simulink model "Ballbot_System_LQR"  (R2020b)
settings: Solver=VariableStepAuto  StartTime=0.0  StopTime=30  RelTol=1e-3
values from neighbouring files (symbols this model uses):
  a_d = 0.8    [SYSTEM_BALLBOT.m]
  a_gc = 0.8    [SYSTEM_BALLBOT.m]
  a_gd = 0.999    [SYSTEM_BALLBOT.m]
  BATTERY = 8000    [SYSTEM_BALLBOT.m]
  GYRO0 = 600    [SYSTEM_BALLBOT.m]
  k_f = K_lqr(1:4)    [SYSTEM_BALLBOT.m]
  pwm_gain = 1    [SYSTEM_BALLBOT.m]
  pwm_offset = 0    [SYSTEM_BALLBOT.m]
  TIME_START = 100    [SYSTEM_BALLBOT.m]
  TS = 0.004    [SYSTEM_BALLBOT.m]
  ts1 = 0.004    [SYSTEM_BALLBOT.m]
  XIV = [ ... (first row only)    [SYSTEM_BALLBOT.m]
undefined symbols (not defined in the file or in its folder): A, B, C, D, Rs, Rw
libraries: legoev3lib x9, simulink x3
settings Model: Creator=ADMIN  LastModifiedBy=ADMIN
settings DebuggingCC: UnconnectedInputMsg=none  UnconnectedOutputMsg=none  UnconnectedLineMsg=none
settings ModelReferenceCC: EnableRefExpFcnMdlSchedulingChecks=off
settings RTWCC: GPUComputeCapability=5.0
settings ConfigComp: CovBoundaryAbsTol=1.0e-5

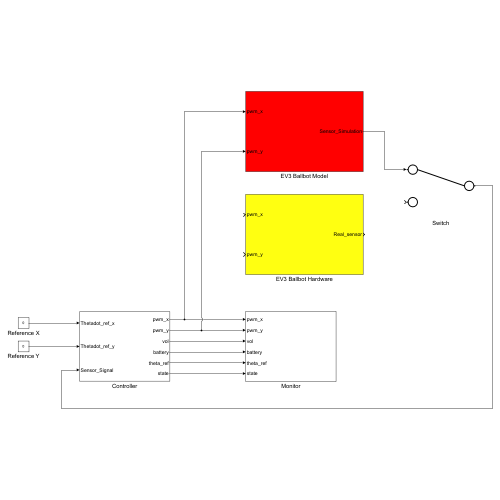
[thumbnail: Simulink's stored preview of the top-level diagram]
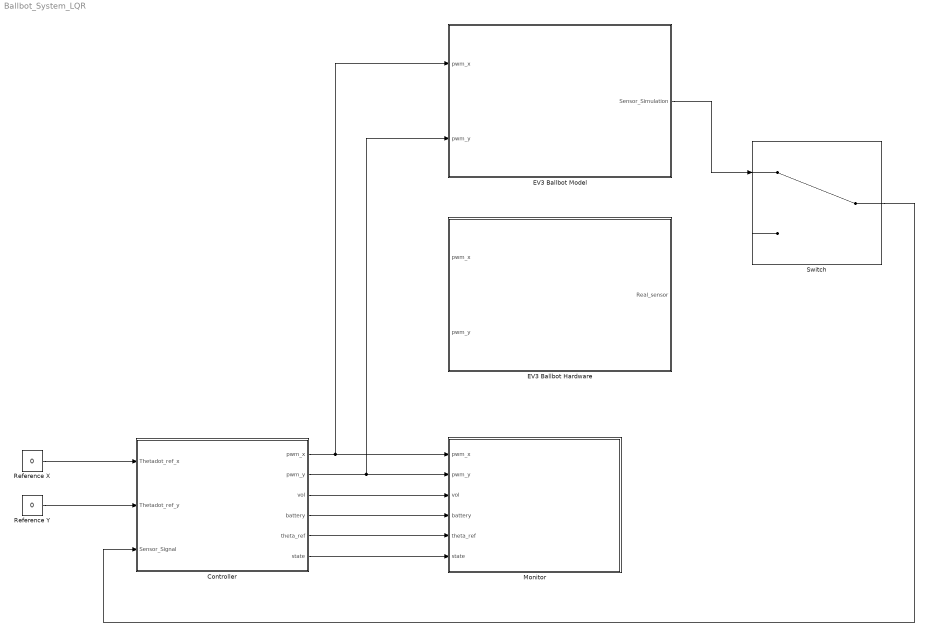
== system Ballbot_System_LQR ==
  Controller : Subsystem
  EV3 Ballbot Hardware : Subsystem
  EV3 Ballbot Model : Subsystem
  Monitor : Subsystem
  Reference X : Constant  Value=0
  Reference Y : Constant  Value=0
  Switch : ManualSwitch
  wires:
  Controller/1(pwm_x) -> EV3 Ballbot Model/1(pwm_x), Monitor/1(pwm_x)
  Controller/4(battery) -> Monitor/4(battery)
  Controller/6(state) -> Monitor/6(state)
  EV3 Ballbot Model/1(Sensor_Simulation) -> Switch/1
  Controller/5(theta_ref) -> Monitor/5(theta_ref)
  Switch/1 -> Controller/3(Sensor_Signal)
  Controller/3(vol) -> Monitor/3(vol)
  Reference Y/1 -> Controller/2(Thetadot_ref_y)
  Controller/2(pwm_y) -> EV3 Ballbot Model/2(pwm_y), Monitor/2(pwm_y)
  Reference X/1 -> Controller/1(Thetadot_ref_x)

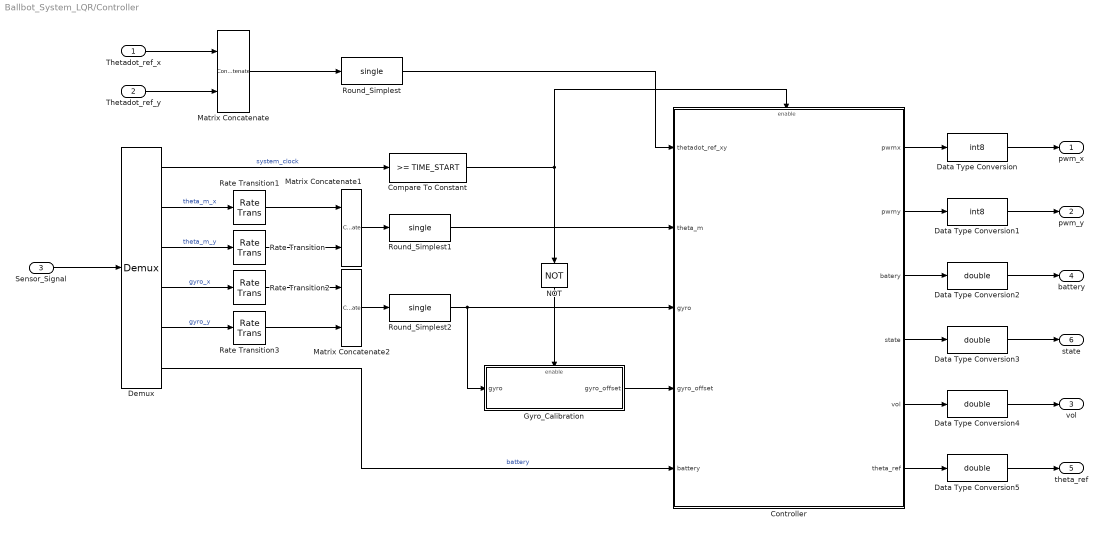
== system Ballbot_System_LQR/Controller ==
  Thetadot_ref_x : Inport
  Thetadot_ref_y : Inport  Port=2
  Sensor_Signal : Inport  Port=3
  Compare To Constant : simulink/Logic and Bit Operations/Compare To Constant  relop=>=  const=TIME_START  OutDataTypeStr=boolean
  Controller : Subsystem
  Data Type Conversion : DataTypeConversion  OutDataTypeStr=int8  RndMeth=Simplest
  Data Type Conversion1 : DataTypeConversion  OutDataTypeStr=int8  RndMeth=Simplest
  Data Type Conversion{2..5} (4 alike) : DataTypeConversion  OutDataTypeStr=double  RndMeth=Simplest
  Demux : Demux  Outputs=6
      settings: DisplayOption=none
  Gyro_Calibration : Subsystem
  Matrix Concatenate : Concatenate  Mode=Multidimensional array  ConcatenateDimension=2
  Matrix Concatenate1 : Concatenate  Mode=Multidimensional array  ConcatenateDimension=2
  Matrix Concatenate2 : Concatenate  Mode=Multidimensional array  ConcatenateDimension=2
  NOT : Logic  Operator=NOT  IconShape=distinctive  AllPortsSameDT=off  OutDataTypeStr=boolean
  Rate Transition{,1..3} (4 alike) : RateTransition  OutPortSampleTime=TS
  Round_Simplest : DataTypeConversion  OutDataTypeStr=single  RndMeth=Round
  Round_Simplest1 : DataTypeConversion  OutDataTypeStr=single  RndMeth=Round
  Round_Simplest2 : DataTypeConversion  OutDataTypeStr=single  RndMeth=Round
  pwm_x : Outport
  pwm_y : Outport  Port=2
  vol : Outport  Port=3
  battery : Outport  Port=4
  theta_ref : Outport  Port=5
  state : Outport  Port=6
  wires:
  Thetadot_ref_x/1 -> Matrix Concatenate/1
  Thetadot_ref_y/1 -> Matrix Concatenate/2
  Matrix Concatenate/1 -> Round_Simplest/1
  Sensor_Signal/1 -> Demux/1
  Demux/3 -> Rate Transition/1  "theta_m_y"
  Matrix Concatenate1/1 -> Round_Simplest1/1
  Matrix Concatenate2/1 -> Round_Simplest2/1
  Demux/1 -> Compare To Constant/1  "system_clock"
  Compare To Constant/1 -> Controller/Enable, NOT/1
  Round_Simplest2/1 -> Controller/3(gyro), Gyro_Calibration/1(gyro)
  NOT/1 -> Gyro_Calibration/Enable
  Demux/6 -> Controller/5(battery)  "battery"
  Gyro_Calibration/1(gyro_offset) -> Controller/4(gyro_offset)
  Round_Simplest1/1 -> Controller/2(theta_m)
  Round_Simplest/1 -> Controller/1(thetadot_ref_xy)
  Controller/1(pwmx) -> Data Type Conversion/1
  Data Type Conversion/1 -> pwm_x/1
  Data Type Conversion1/1 -> pwm_y/1
  Controller/2(pwmy) -> Data Type Conversion1/1
  Data Type Conversion2/1 -> battery/1
  Controller/3(batery) -> Data Type Conversion2/1
  Data Type Conversion3/1 -> state/1
  Controller/4(state) -> Data Type Conversion3/1
  Data Type Conversion4/1 -> vol/1
  Controller/5(vol) -> Data Type Conversion4/1
  Data Type Conversion5/1 -> theta_ref/1
  Controller/6(theta_ref) -> Data Type Conversion5/1
  Rate Transition/1 -> Matrix Concatenate1/2
  Rate Transition1/1 -> Matrix Concatenate1/1
  Demux/4 -> Rate Transition2/1  "gyro_x"
  Rate Transition2/1 -> Matrix Concatenate2/1
  Demux/2 -> Rate Transition1/1  "theta_m_x"
  Rate Transition3/1 -> Matrix Concatenate2/2
  Demux/5 -> Rate Transition3/1  "gyro_y"

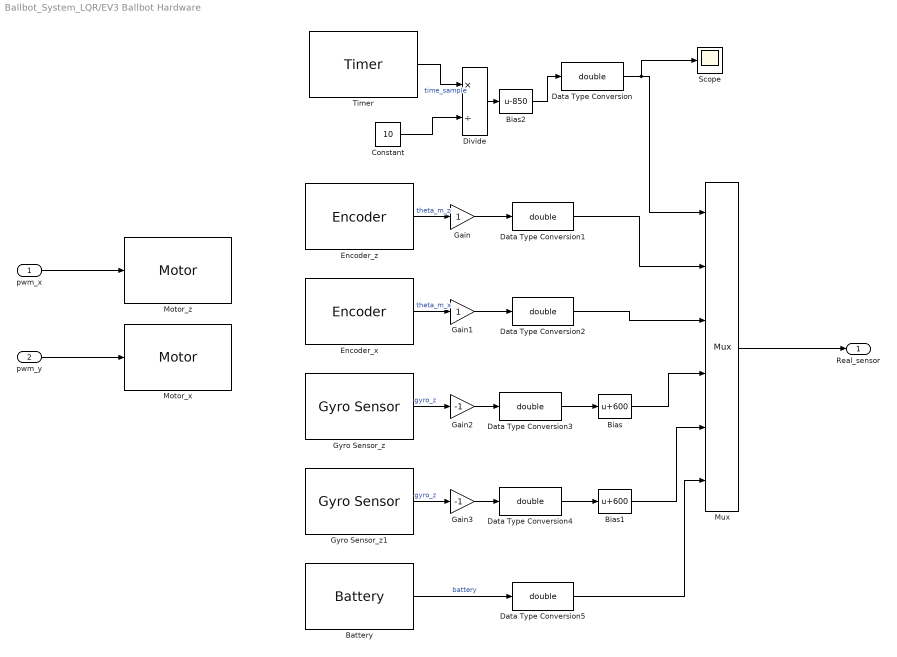
== system Ballbot_System_LQR/EV3 Ballbot Hardware ==
  pwm_x : Inport
  pwm_y : Inport  Port=2
  Battery : legoev3lib/Battery  SampleTime=TS
  Bias : Bias  Bias=600
  Bias1 : Bias  Bias=600
  Bias2 : Bias  Bias=-850
  Constant : Constant  Value=10
  Data Type Conversion{,1..5} (6 alike) : DataTypeConversion  OutDataTypeStr=double  RndMeth=Nearest
  Divide : Product  Inputs=*/
  Encoder_x : legoev3lib/Encoder  portNumber=C  opMode=Reset by external signal  sampleTime=TS
  Encoder_z : legoev3lib/Encoder  portNumber=B  opMode=Reset by external signal  sampleTime=TS
  Gain : Gain
  Gain1 : Gain
  Gain2 : Gain  Gain=-1
  Gain3 : Gain  Gain=-1
  Gyro Sensor_z : legoev3lib/Gyro Sensor  portNumber=2  sampleTime=TS
  Gyro Sensor_z1 : legoev3lib/Gyro Sensor  portNumber=3  sampleTime=TS
  Motor_x : legoev3lib/Motor  sportNumber=C  sstopAction=Brake
  Motor_z : legoev3lib/Motor  sportNumber=B  sstopAction=Brake
  Mux : Mux  Inputs=6
      settings: DisplayOption=signals
  Scope : Scope
  Timer : legoev3lib/Timer  SampleTime=TS
  Real_sensor : Outport
  wires:
  pwm_x/1 -> Motor_z/1
  pwm_y/1 -> Motor_x/1
  Timer/1 -> Divide/1  "time_sample"
  Encoder_z/1 -> Gain/1  "theta_m_z"
  Encoder_x/1 -> Gain1/1  "theta_m_x"
  Battery/1 -> Data Type Conversion5/1  "battery"
  Data Type Conversion/1 -> Scope/1, Mux/1
  Data Type Conversion1/1 -> Mux/2
  Data Type Conversion2/1 -> Mux/3
  Data Type Conversion5/1 -> Mux/6
  Mux/1 -> Real_sensor/1
  Gain/1 -> Data Type Conversion1/1
  Gain1/1 -> Data Type Conversion2/1
  Gain2/1 -> Data Type Conversion3/1
  Gyro Sensor_z/1 -> Gain2/1  "gyro_z"
  Gyro Sensor_z1/1 -> Gain3/1  "gyro_z"
  Gain3/1 -> Data Type Conversion4/1
  Data Type Conversion3/1 -> Bias/1
  Data Type Conversion4/1 -> Bias1/1
  Bias/1 -> Mux/4
  Bias1/1 -> Mux/5
  Constant/1 -> Divide/2
  Divide/1 -> Bias2/1
  Bias2/1 -> Data Type Conversion/1

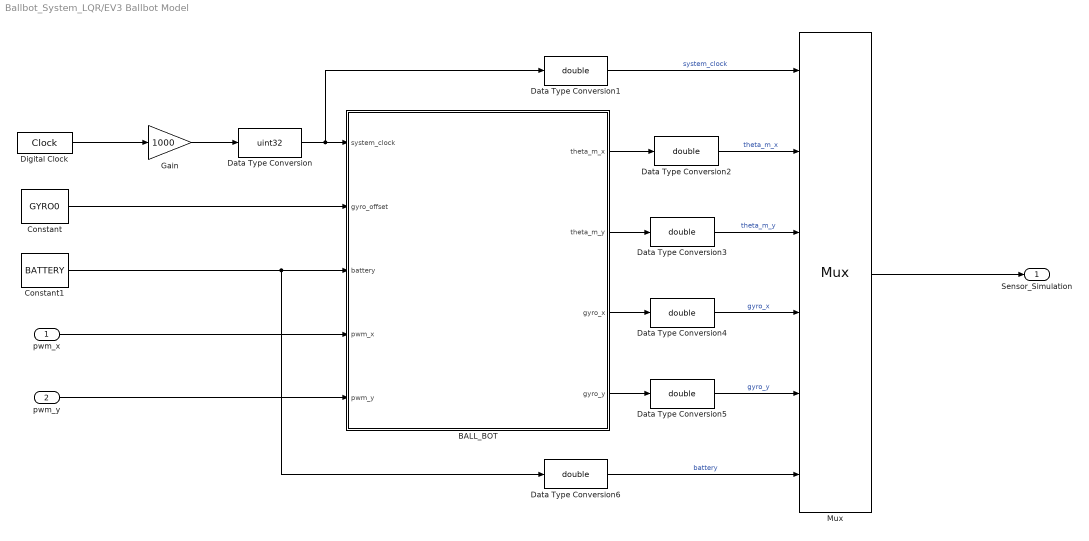
== system Ballbot_System_LQR/EV3 Ballbot Model ==
  pwm_x : Inport
  pwm_y : Inport  Port=2
  BALL_BOT : Subsystem
  Constant : Constant  Value=GYRO0  OutDataTypeStr=uint16
  Constant1 : Constant  Value=BATTERY  OutDataTypeStr=uint16
  Data Type Conversion : DataTypeConversion  OutDataTypeStr=uint32  RndMeth=Nearest
  Data Type Conversion{1..6} (6 alike) : DataTypeConversion  OutDataTypeStr=double  RndMeth=Nearest
  Digital Clock : DigitalClock
  Gain : Gain  Gain=1000
  Mux : Mux  Inputs=6
      settings: DisplayOption=signals
  Sensor_Simulation : Outport
  wires:
  Digital Clock/1 -> Gain/1
  Gain/1 -> Data Type Conversion/1
  Data Type Conversion/1 -> Data Type Conversion1/1, BALL_BOT/1(system_clock)
  Constant/1 -> BALL_BOT/2(gyro_offset)
  Constant1/1 -> Data Type Conversion6/1, BALL_BOT/3(battery)
  pwm_x/1 -> BALL_BOT/4(pwm_x)
  pwm_y/1 -> BALL_BOT/5(pwm_y)
  BALL_BOT/1(theta_m_x) -> Data Type Conversion2/1
  BALL_BOT/2(theta_m_y) -> Data Type Conversion3/1
  BALL_BOT/3(gyro_x) -> Data Type Conversion4/1
  BALL_BOT/4(gyro_y) -> Data Type Conversion5/1
  Data Type Conversion1/1 -> Mux/1  "system_clock"
  Data Type Conversion2/1 -> Mux/2  "theta_m_x"
  Data Type Conversion3/1 -> Mux/3  "theta_m_y"
  Data Type Conversion4/1 -> Mux/4  "gyro_x"
  Data Type Conversion5/1 -> Mux/5  "gyro_y"
  Data Type Conversion6/1 -> Mux/6  "battery"
  Mux/1 -> Sensor_Simulation/1

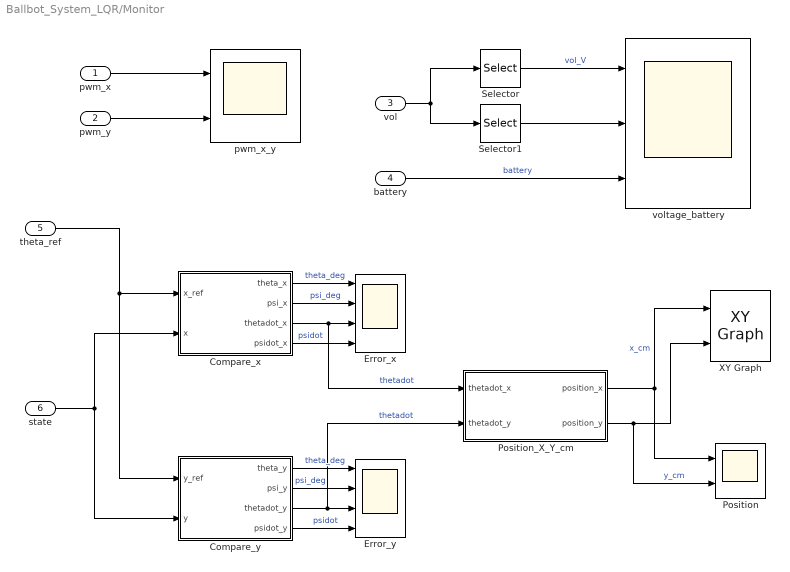
== system Ballbot_System_LQR/Monitor ==
  pwm_x : Inport
  pwm_y : Inport  Port=2
  vol : Inport  Port=3
  battery : Inport  Port=4
  theta_ref : Inport  Port=5
  state : Inport  Port=6
  Compare_x : Subsystem
  Compare_y : Subsystem
  Error_x : Scope  NumInputPorts=4
  Error_y : Scope  NumInputPorts=4
  Position : Scope  NumInputPorts=2
  Position_X_Y_cm : Subsystem
  Selector : Selector  InputPortWidth=2  IndexOptions=Index vector (dialog)  Indices=1  OutputSizes=1
  Selector1 : Selector  InputPortWidth=2  IndexOptions=Index vector (dialog)  Indices=2  OutputSizes=1
  XY Graph : simulink/Sinks/XY Graph  xmin=-1  xmax=1  ymin=-1  ymax=1  st=-1
  pwm_x_y : Scope  NumInputPorts=2
  voltage_battery : Scope  NumInputPorts=3
  wires:
  pwm_x/1 -> pwm_x_y/1
  pwm_y/1 -> pwm_x_y/2
  Selector/1 -> voltage_battery/1  "vol_V"
  Selector1/1 -> voltage_battery/2
  vol/1 -> Selector/1, Selector1/1
  battery/1 -> voltage_battery/3  "battery"
  state/1 -> Compare_y/2(y), Compare_x/2(x)
  Compare_x/1(theta_x) -> Error_x/1  "theta_deg"
  Compare_x/2(psi_x) -> Error_x/2  "psi_deg"
  Compare_x/3(thetadot_x) -> Error_x/3, Position_X_Y_cm/1(thetadot_x)  "thetadot"
  Compare_x/4(psidot_x) -> Error_x/4  "psidot"
  Compare_y/2(psi_y) -> Error_y/2  "psi_deg"
  Compare_y/1(theta_y) -> Error_y/1  "theta_deg"
  Compare_y/3(thetadot_y) -> Position_X_Y_cm/2(thetadot_y), Error_y/3  "thetadot"
  Compare_y/4(psidot_y) -> Error_y/4  "psidot"
  theta_ref/1 -> Compare_y/1(y_ref), Compare_x/1(x_ref)
  Position_X_Y_cm/1(position_x) -> Position/1, XY Graph/1  "x_cm"
  Position_X_Y_cm/2(position_y) -> Position/2, XY Graph/2  "y_cm"

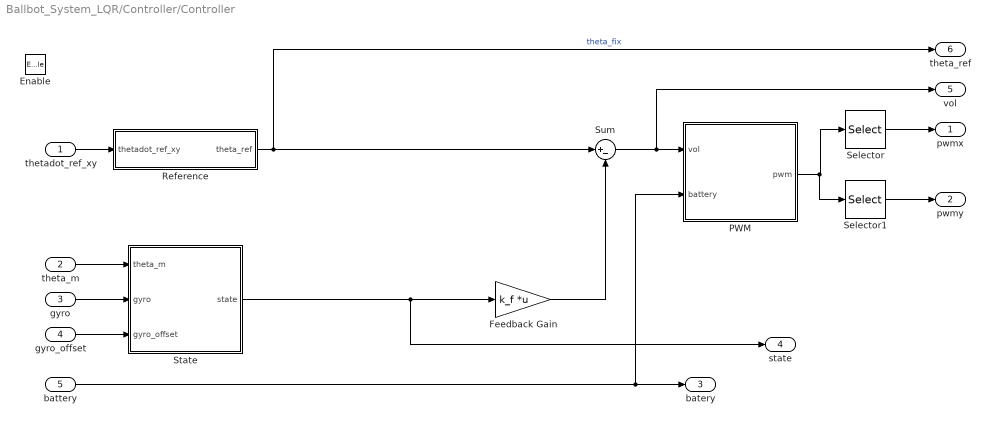
== system Ballbot_System_LQR/Controller/Controller ==
  thetadot_ref_xy : Inport
  theta_m : Inport  Port=2
  gyro : Inport  Port=3
  gyro_offset : Inport  Port=4
  battery : Inport  Port=5
  Enable : EnablePort
  Feedback Gain : Gain  Gain=k_f  Multiplication=Matrix(K*u)  OutDataTypeStr=Inherit: Same as input  ParamDataTypeStr=Inherit: Same as input
  PWM : Subsystem
  Reference : Subsystem
  Selector : Selector  InputPortWidth=2  IndexOptions=Index vector (dialog)  Indices=1  OutputSizes=1
  Selector1 : Selector  InputPortWidth=2  IndexOptions=Index vector (dialog)  Indices=2  OutputSizes=1
  State : Subsystem
  Sum : Sum  Inputs=|+-  OutDataTypeStr=Inherit: Same as first input
  pwmx : Outport
  pwmy : Outport  Port=2
  batery : Outport  Port=3
  state : Outport  Port=4
  vol : Outport  Port=5
  theta_ref : Outport  Port=6
  wires:
  Feedback Gain/1 -> Sum/2
  Sum/1 -> vol/1, PWM/1(vol)
  gyro_offset/1 -> State/3(gyro_offset)
  thetadot_ref_xy/1 -> Reference/1(thetadot_ref_xy)
  battery/1 -> batery/1, PWM/2(battery)
  theta_m/1 -> State/1(theta_m)
  State/1(state) -> state/1, Feedback Gain/1
  gyro/1 -> State/2(gyro)
  PWM/1(pwm) -> Selector1/1, Selector/1
  Selector/1 -> pwmx/1
  Selector1/1 -> pwmy/1
  Reference/1(theta_ref) -> theta_ref/1, Sum/1  "theta_fix"

== system Ballbot_System_LQR/Controller/Gyro_Calibration ==
  note: Low Path Filter
      |   gyro_offset = (1 - a_gc) * gyro_read + a_gc * gyro_offset
  gyro : Inport
  Enable : EnablePort
  Freq : Constant  Value=440
  Gain : Gain  Gain=1-a_gc
  Gain1 : Gain  Gain=a_gc
  Speaker : legoev3lib/Speaker  sinputMode=Frequency only  sspeakerFreq=100  sspeakerVolume=50  sspeakerDuration=100
  Sum : Sum  Inputs=|++
  Unit Delay : UnitDelay  SampleTime=-1  HasFrameUpgradeWarning=on
  gyro_offset : Outport
  wires:
  Freq/1 -> Speaker/1
  gyro/1 -> Gain/1
  Gain/1 -> Sum/1
  Gain1/1 -> Sum/2
  Unit Delay/1 -> Gain1/1
  Sum/1 -> Unit Delay/1, gyro_offset/1

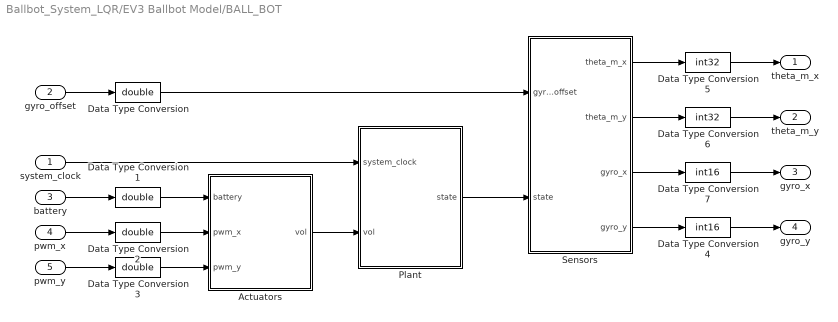
== system Ballbot_System_LQR/EV3 Ballbot Model/BALL_BOT ==
  system_clock : Inport
  gyro_offset : Inport  Port=2
  battery : Inport  Port=3
  pwm_x : Inport  Port=4
  pwm_y : Inport  Port=5
  Actuators : Subsystem
  Data Type Conversion{,1..3} (4 alike) : DataTypeConversion  OutDataTypeStr=double  RndMeth=Nearest
      settings: AttributesFormatString=Round = %<RndMeth>
  Data Type Conversion4 : DataTypeConversion  OutDataTypeStr=int16  RndMeth=Nearest
      settings: AttributesFormatString=Round = %<RndMeth>
  Data Type Conversion5 : DataTypeConversion  OutDataTypeStr=int32  RndMeth=Nearest
      settings: AttributesFormatString=Round = %<RndMeth>
  Data Type Conversion6 : DataTypeConversion  OutDataTypeStr=int32  RndMeth=Nearest
      settings: AttributesFormatString=Round = %<RndMeth>
  Data Type Conversion7 : DataTypeConversion  OutDataTypeStr=int16  RndMeth=Nearest
      settings: AttributesFormatString=Round = %<RndMeth>
  Plant : Subsystem
  Sensors : Subsystem
  theta_m_x : Outport
  theta_m_y : Outport  Port=2
  gyro_x : Outport  Port=3
  gyro_y : Outport  Port=4
  wires:
  Data Type Conversion6/1 -> theta_m_y/1
  Data Type Conversion2/1 -> Actuators/2(pwm_x)
  system_clock/1 -> Plant/1(system_clock)
  gyro_offset/1 -> Data Type Conversion/1
  Data Type Conversion5/1 -> theta_m_x/1
  pwm_y/1 -> Data Type Conversion3/1
  pwm_x/1 -> Data Type Conversion2/1
  Data Type Conversion3/1 -> Actuators/3(pwm_y)
  battery/1 -> Data Type Conversion1/1
  Data Type Conversion1/1 -> Actuators/1(battery)
  Actuators/1(vol) -> Plant/2(vol)
  Data Type Conversion7/1 -> gyro_x/1
  Data Type Conversion/1 -> Sensors/1(gyro_offset)
  Plant/1(state) -> Sensors/2(state)
  Sensors/4(gyro_y) -> Data Type Conversion4/1
  Data Type Conversion4/1 -> gyro_y/1
  Sensors/3(gyro_x) -> Data Type Conversion7/1
  Sensors/2(theta_m_y) -> Data Type Conversion6/1
  Sensors/1(theta_m_x) -> Data Type Conversion5/1

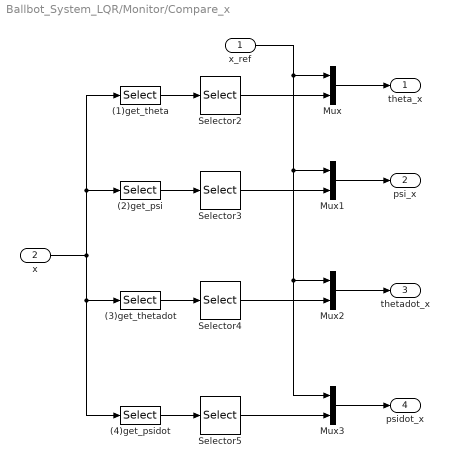
== system Ballbot_System_LQR/Monitor/Compare_x ==
  x_ref : Inport
  x : Inport  Port=2
  (1)get_theta : Selector  NumberOfDimensions=2  InputPortWidth=2  IndexOptions=Index vector (dialog),Index vector (dialog)  Indices=1,[1,2]  OutputSizes=1,1
  (2)get_psi : Selector  NumberOfDimensions=2  InputPortWidth=2  IndexOptions=Index vector (dialog),Index vector (dialog)  Indices=2,[1,2]  OutputSizes=1,1
  (3)get_thetadot : Selector  NumberOfDimensions=2  InputPortWidth=2  IndexOptions=Index vector (dialog),Index vector (dialog)  Indices=3,[1,2]  OutputSizes=1,1
  (4)get_psidot : Selector  NumberOfDimensions=2  InputPortWidth=2  IndexOptions=Index vector (dialog),Index vector (dialog)  Indices=4,[1,2]  OutputSizes=1,1
  Mux{,1..3} (4 alike) : Mux  Inputs=2
  Selector{2..5} (4 alike) : Selector  InputPortWidth=2  IndexOptions=Index vector (dialog)  Indices=1  OutputSizes=1
  theta_x : Outport
  psi_x : Outport  Port=2
  thetadot_x : Outport  Port=3
  psidot_x : Outport  Port=4
  wires:
  (1)get_theta/1 -> Selector2/1
  x/1 -> (3)get_thetadot/1, (4)get_psidot/1, (2)get_psi/1, (1)get_theta/1
  (2)get_psi/1 -> Selector3/1
  (3)get_thetadot/1 -> Selector4/1
  (4)get_psidot/1 -> Selector5/1
  x_ref/1 -> Mux3/1, Mux2/1, Mux1/1, Mux/1
  Selector2/1 -> Mux/2
  Mux/1 -> theta_x/1
  Selector3/1 -> Mux1/2
  Mux1/1 -> psi_x/1
  Selector4/1 -> Mux2/2
  Mux2/1 -> thetadot_x/1
  Selector5/1 -> Mux3/2
  Mux3/1 -> psidot_x/1

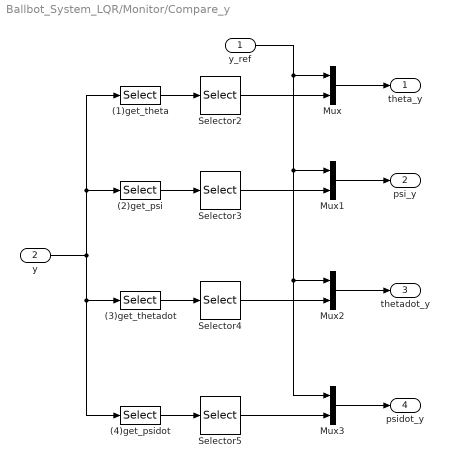
== system Ballbot_System_LQR/Monitor/Compare_y ==
  y_ref : Inport
  y : Inport  Port=2
  (1)get_theta : Selector  NumberOfDimensions=2  InputPortWidth=2  IndexOptions=Index vector (dialog),Index vector (dialog)  Indices=1,[1,2]  OutputSizes=1,1
  (2)get_psi : Selector  NumberOfDimensions=2  InputPortWidth=2  IndexOptions=Index vector (dialog),Index vector (dialog)  Indices=2,[1,2]  OutputSizes=1,1
  (3)get_thetadot : Selector  NumberOfDimensions=2  InputPortWidth=2  IndexOptions=Index vector (dialog),Index vector (dialog)  Indices=3,[1,2]  OutputSizes=1,1
  (4)get_psidot : Selector  NumberOfDimensions=2  InputPortWidth=2  IndexOptions=Index vector (dialog),Index vector (dialog)  Indices=4,[1,2]  OutputSizes=1,1
  Mux{,1..3} (4 alike) : Mux  Inputs=2
  Selector{2..5} (4 alike) : Selector  InputPortWidth=2  IndexOptions=Index vector (dialog)  Indices=2  OutputSizes=1
  theta_y : Outport
  psi_y : Outport  Port=2
  thetadot_y : Outport  Port=3
  psidot_y : Outport  Port=4
  wires:
  y_ref/1 -> Mux3/1, Mux2/1, Mux1/1, Mux/1
  Selector4/1 -> Mux2/2
  Mux2/1 -> thetadot_y/1
  Selector5/1 -> Mux3/2
  Mux/1 -> theta_y/1
  (4)get_psidot/1 -> Selector5/1
  (3)get_thetadot/1 -> Selector4/1
  (2)get_psi/1 -> Selector3/1
  y/1 -> (3)get_thetadot/1, (4)get_psidot/1, (2)get_psi/1, (1)get_theta/1
  Selector3/1 -> Mux1/2
  Mux1/1 -> psi_y/1
  (1)get_theta/1 -> Selector2/1
  Mux3/1 -> psidot_y/1
  Selector2/1 -> Mux/2

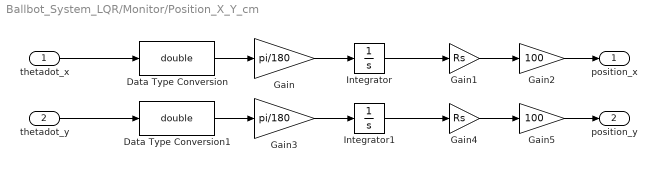
== system Ballbot_System_LQR/Monitor/Position_X_Y_cm ==
  thetadot_x : Inport
  thetadot_y : Inport  Port=2
  Data Type Conversion : DataTypeConversion  OutDataTypeStr=double  RndMeth=Nearest
  Data Type Conversion1 : DataTypeConversion  OutDataTypeStr=double  RndMeth=Nearest
  Gain : Gain  Gain=pi/180
  Gain1 : Gain  Gain=Rs
  Gain2 : Gain  Gain=100
  Gain3 : Gain  Gain=pi/180
  Gain4 : Gain  Gain=Rs
  Gain5 : Gain  Gain=100
  Integrator : Integrator
  Integrator1 : Integrator
  position_x : Outport
  position_y : Outport  Port=2
  wires:
  thetadot_x/1 -> Data Type Conversion/1
  Data Type Conversion/1 -> Gain/1
  Gain/1 -> Integrator/1
  Integrator/1 -> Gain1/1
  Gain1/1 -> Gain2/1
  Gain2/1 -> position_x/1
  Gain3/1 -> Integrator1/1
  Gain4/1 -> Gain5/1
  Gain5/1 -> position_y/1
  thetadot_y/1 -> Data Type Conversion1/1
  Integrator1/1 -> Gain4/1
  Data Type Conversion1/1 -> Gain3/1

== system Ballbot_System_LQR/Controller/Controller/PWM ==
  note: Calculate maximum of DC motor
      | voltatege from the battery using
      | the experimental expression.
  note: Compensate coulombic and
      | viscous friction of the drive system
  vol : Inport
  battery : Inport  Port=2
  Cal_vol_max : Subsystem
  Friction Compensator : simulink/Discontinuities/Coulomb & Viscous Friction  offset=pwm_offset  gain=pwm_gain
      settings: AttributesFormatString=gain = %<gain>\noffset = %<offset>
  Gain : Gain  Gain=100  OutDataTypeStr=Inherit: Same as input  ParamDataTypeStr=Inherit: Same as input
  Product : Product  Inputs=*/  RndMeth=Simplest  OutDataTypeStr=Inherit: Same as first input
  Saturation : Saturate  UpperLimit=100  LowerLimit=-100
      settings: AttributesFormatString=max = %<UpperLimit>\nmin = %<LowerLimit>
  pwm : Outport
  wires:
  Gain/1 -> Friction Compensator/1
  Saturation/1 -> pwm/1
  vol/1 -> Product/1
  Product/1 -> Gain/1
  battery/1 -> Cal_vol_max/1(battery)
  Cal_vol_max/1(vol_max) -> Product/2
  Friction Compensator/1 -> Saturation/1

== system Ballbot_System_LQR/Controller/Controller/Reference ==
  thetadot_ref_xy : Inport
  Discrete Integrator : Subsystem
  Integrator : Integrator
  theta_ref : Outport
  wires:
  thetadot_ref_xy/1 -> Discrete Integrator/1(in)
  Discrete Integrator/1(out) -> theta_ref/1

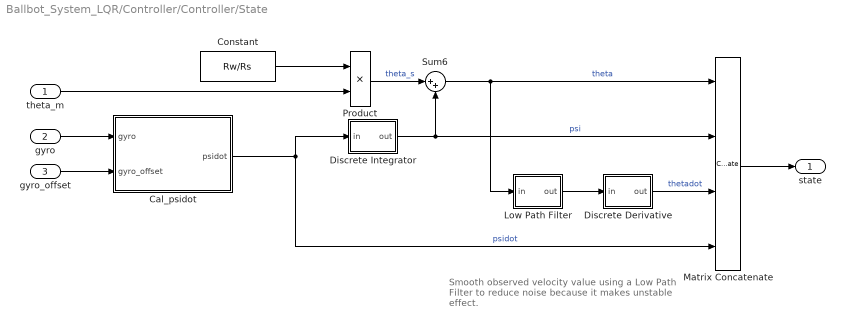
== system Ballbot_System_LQR/Controller/Controller/State ==
  note: Smooth observed velocity value using
      | a Low Path Filter to reduce noise
      | because it makes unstable effect.
  theta_m : Inport
  gyro : Inport  Port=2
  gyro_offset : Inport  Port=3
  Cal_psidot : Subsystem
  Constant : Constant  Value=Rw/Rs  OutDataTypeStr=single
  Discrete Derivative : Subsystem
  Discrete Integrator : Subsystem
  Low Path Filter : Subsystem
  Matrix Concatenate : Concatenate  NumInputs=4  Mode=Multidimensional array
  Product : Product  RndMeth=Simplest  OutDataTypeStr=Inherit: Same as first input
  Sum6 : Sum  Inputs=|++  OutDataTypeStr=Inherit: Same as first input
  state : Outport
  wires:
  Discrete Integrator/1(out) -> Sum6/2, Matrix Concatenate/2  "psi"
  theta_m/1 -> Product/2
  Discrete Derivative/1(out) -> Matrix Concatenate/3  "thetadot"
  Sum6/1 -> Low Path Filter/1(in), Matrix Concatenate/1  "theta"
  gyro/1 -> Cal_psidot/1(gyro)
  Low Path Filter/1(out) -> Discrete Derivative/1(in)
  Product/1 -> Sum6/1  "theta_s"
  Matrix Concatenate/1 -> state/1
  Cal_psidot/1(psidot) -> Discrete Integrator/1(in), Matrix Concatenate/4  "psidot"
  gyro_offset/1 -> Cal_psidot/2(gyro_offset)
  Constant/1 -> Product/1

== system Ballbot_System_LQR/EV3 Ballbot Model/BALL_BOT/Actuators ==
  note: Dead zone of drive system
  note: Calculate maximum of DC motor voltatege from
      | battery using an experimental expression.
  battery : Inport
  pwm_x : Inport  Port=2
  pwm_y : Inport  Port=3
  Cal_vol_max : Subsystem
  Dead Zone : DeadZone  LowerValue=-pwm_offset  UpperValue=pwm_offset  SaturateOnIntegerOverflow=on
      settings: AttributesFormatString=start=%<LowerValue>\nend=%<UpperValue>
  Gain1 : Gain  Gain=1/pwm_gain  OutDataTypeStr=Inherit: Same as input  ParamDataTypeStr=Inherit: Same as input
  Gain2 : Gain  Gain=1/100  OutDataTypeStr=Inherit: Same as input  ParamDataTypeStr=Inherit: Same as input
  Matrix Concatenate1 : Concatenate  Mode=Multidimensional array  ConcatenateDimension=2
  Product : Product  RndMeth=Simplest
  vol : Outport
  wires:
  Gain1/1 -> Gain2/1
  Gain2/1 -> Product/1
  Product/1 -> vol/1
  Dead Zone/1 -> Gain1/1
  Cal_vol_max/1(vol_max) -> Product/2
  battery/1 -> Cal_vol_max/1(battery)
  pwm_x/1 -> Matrix Concatenate1/1
  pwm_y/1 -> Matrix Concatenate1/2
  Matrix Concatenate1/1 -> Dead Zone/1

== system Ballbot_System_LQR/EV3 Ballbot Model/BALL_BOT/Plant ==
  note: Start plant calculation after gyro calibration.
      | (TIME_START is calibration time)
  system_clock : Inport
  vol : Inport  Port=2
  Constant : Constant  Value=TIME_START  OutDataTypeStr=uint32
      settings: AttributesFormatString=DataType = %<OutDataTypeStr>
  Enabled Subsystem : Subsystem  TreatAsAtomicUnit=on
  Relational Operator : RelationalOperator  OutDataTypeStr=boolean  RndMeth=Nearest
  state : Outport
  wires:
  vol/1 -> Enabled Subsystem/1(vol)
  Relational Operator/1 -> Enabled Subsystem/Enable
  system_clock/1 -> Relational Operator/1
  Constant/1 -> Relational Operator/2
  Enabled Subsystem/1(state) -> state/1

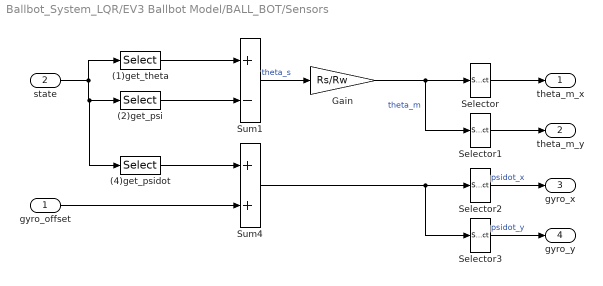
== system Ballbot_System_LQR/EV3 Ballbot Model/BALL_BOT/Sensors ==
  gyro_offset : Inport
  state : Inport  Port=2
  (1)get_theta : Selector  NumberOfDimensions=2  InputPortWidth=2  IndexOptions=Index vector (dialog),Index vector (dialog)  Indices=1,[1,2]  OutputSizes=1,1
  (2)get_psi : Selector  NumberOfDimensions=2  InputPortWidth=2  IndexOptions=Index vector (dialog),Index vector (dialog)  Indices=2,[1,2]  OutputSizes=1,1
  (4)get_psidot : Selector  NumberOfDimensions=2  InputPortWidth=2  IndexOptions=Index vector (dialog),Index vector (dialog)  Indices=4,[1,2]  OutputSizes=1,1
  Gain : Gain  Gain=Rs/Rw
  Selector : Selector  InputPortWidth=2  IndexOptions=Index vector (dialog)  Indices=1  OutputSizes=1
  Selector1 : Selector  InputPortWidth=2  IndexOptions=Index vector (dialog)  Indices=2  OutputSizes=1
  Selector2 : Selector  InputPortWidth=2  IndexOptions=Index vector (dialog)  Indices=1  OutputSizes=1
  Selector3 : Selector  InputPortWidth=2  IndexOptions=Index vector (dialog)  Indices=2  OutputSizes=1
  Sum1 : Sum  Inputs=+-
  Sum4 : Sum
  theta_m_x : Outport
  theta_m_y : Outport  Port=2
  gyro_x : Outport  Port=3
  gyro_y : Outport  Port=4
  wires:
  Sum1/1 -> Gain/1  "theta_s"
  Gain/1 -> Selector/1, Selector1/1  "theta_m"
  Selector/1 -> theta_m_x/1
  Selector1/1 -> theta_m_y/1
  Sum4/1 -> Selector2/1, Selector3/1
  Selector2/1 -> gyro_x/1  "psidot_x"
  Selector3/1 -> gyro_y/1  "psidot_y"
  (1)get_theta/1 -> Sum1/1
  (2)get_psi/1 -> Sum1/2
  state/1 -> (4)get_psidot/1, (2)get_psi/1, (1)get_theta/1
  (4)get_psidot/1 -> Sum4/1
  gyro_offset/1 -> Sum4/2

== system Ballbot_System_LQR/Controller/Controller/PWM/Cal_vol_max ==
  battery : Inport
  Constant : Constant  Value=0.625  OutDataTypeStr=single  SampleTime=-1
      settings: AttributesFormatString=DataType = %<OutDataTypeStr>
  Gain3 : Gain  Gain=0.001089  OutDataTypeStr=Inherit: Same as input  ParamDataTypeStr=Inherit: Same as input
  Sum2 : Sum  Inputs=|+-  OutDataTypeStr=Inherit: Same as first input
  vol_max : Outport
  wires:
  Constant/1 -> Sum2/2
  Sum2/1 -> vol_max/1
  Gain3/1 -> Sum2/1
  battery/1 -> Gain3/1

== system Ballbot_System_LQR/Controller/Controller/Reference/Discrete Integrator ==
  note: S(0) = 0
      | S(n) = S(n - 1) + u(n)
      | y(n) = ts1 * S(n) / 1000    (ts1 [msec])
  note: Discrete Integrator (Forward Euler Method)
  in : Inport
  Gain : Gain  Gain=ts1
  Sum : Sum  Inputs=|++
  Unit Delay : UnitDelay  SampleTime=-1  HasFrameUpgradeWarning=on
  out : Outport
  wires:
  Sum/1 -> Unit Delay/1
  in/1 -> Sum/1
  Gain/1 -> out/1
  Unit Delay/1 -> Sum/2, Gain/1

== system Ballbot_System_LQR/Controller/Controller/State/Cal_psidot ==
  gyro : Inport
  gyro_offset : Inport  Port=2
  Sum2 : Sum  Inputs=|+-  OutDataTypeStr=Inherit: Same as first input
  Update_gyro_offset : Subsystem
  psidot : Outport
  wires:
  gyro/1 -> Update_gyro_offset/1(gyro), Sum2/1
  Update_gyro_offset/1(gyro_offset_u) -> Sum2/2
  Sum2/1 -> psidot/1
  gyro_offset/1 -> Update_gyro_offset/2(gyro_offset)

== system Ballbot_System_LQR/Controller/Controller/State/Discrete Derivative ==
  note: u(0) = 0
      | y(n) = 1000 * [u(n) - u(n - 1)] / ts1   (ts1 [msec])
  note: Discrete Derivative (Backward Difference Method)
  in : Inport
  Gain : Gain  Gain=1/ts1
  Sum : Sum  Inputs=|+-
  Unit Delay : UnitDelay  SampleTime=-1  HasFrameUpgradeWarning=on
  out : Outport
  wires:
  in/1 -> Unit Delay/1, Sum/1
  Unit Delay/1 -> Sum/2
  Sum/1 -> Gain/1
  Gain/1 -> out/1

== system Ballbot_System_LQR/Controller/Controller/State/Discrete Integrator ==
  note: S(0) = 0
      | S(n) = S(n - 1) + u(n)
      | y(n) = ts1 * S(n) / 1000    (ts1 [msec])
  note: Discrete Integrator (Forward Euler Method)
  in : Inport
  Gain : Gain  Gain=ts1
  Sum : Sum  Inputs=|++
  Unit Delay : UnitDelay  SampleTime=-1  HasFrameUpgradeWarning=on
  out : Outport
  wires:
  Sum/1 -> Unit Delay/1
  in/1 -> Sum/1
  Gain/1 -> out/1
  Unit Delay/1 -> Sum/2, Gain/1

== system Ballbot_System_LQR/Controller/Controller/State/Low Path Filter ==
  note: Y(z) = H(z) * U(z)
      |                   1 - a
      | H(z) =  -----------------
      |              1 - a * z^(-1)
  note: Low Path Filter
  note: y(0) = 0
      | y(n) = a * y(n - 1) + (1 - a) * u(n)
  in : Inport
  Constant1 : Constant  Value=a_d  VectorParams1D=off  OutDataTypeStr=single  SampleTime=-1
      settings: AttributesFormatString=DataType = %<OutDataTypeStr>
  Constant2 : Constant  VectorParams1D=off  OutDataTypeStr=single  SampleTime=-1
      settings: AttributesFormatString=DataType = %<OutDataTypeStr>
  Product : Product  RndMeth=Simplest  OutDataTypeStr=Inherit: Same as first input
  Product1 : Product  RndMeth=Simplest  OutDataTypeStr=Inherit: Same as first input
  Sum : Sum  Inputs=|++  OutDataTypeStr=Inherit: Same as first input
  Sum1 : Sum  Inputs=|+-  OutDataTypeStr=Inherit: Same as first input
  Unit Delay : UnitDelay  SampleTime=-1  StateName=ud_lpf_theta
      settings: AttributesFormatString=Initial = %<X0>\nState = %<StateIdentifier>
  out : Outport
  wires:
  Sum1/1 -> Product/2
  Unit Delay/1 -> Product1/1
  in/1 -> Product/1
  Product/1 -> Sum/1
  Constant2/1 -> Sum1/1
  Constant1/1 -> Sum1/2, Product1/2
  Sum/1 -> Unit Delay/1, out/1
  Product1/1 -> Sum/2

== system Ballbot_System_LQR/EV3 Ballbot Model/BALL_BOT/Actuators/Cal_vol_max ==
  battery : Inport
  Constant : Constant  Value=0.625  OutDataTypeStr=double
      settings: AttributesFormatString=DataType = %<OutDataTypeStr>
  Gain3 : Gain  Gain=0.001089  OutDataTypeStr=Inherit: Same as input  ParamDataTypeStr=Inherit: Same as input
  Sum2 : Sum  Inputs=|+-  OutDataTypeStr=Inherit: Same as first input
  vol_max : Outport
  wires:
  battery/1 -> Gain3/1
  Gain3/1 -> Sum2/1
  Sum2/1 -> vol_max/1
  Constant/1 -> Sum2/2

== system Ballbot_System_LQR/EV3 Ballbot Model/BALL_BOT/Plant/Enabled Subsystem ==
  note: NXT Ballbot Plant
  note: The linearized model of inverted pendulum in x and y directions.
  vol : Inport  OutDataTypeStr=double
  Enable : EnablePort
  Matrix Concatenate1 : Concatenate  Mode=Multidimensional array  ConcatenateDimension=2
  Selector3 : Selector  InputPortWidth=2  IndexOptions=Index vector (dialog)  Indices=1  OutputSizes=1
  Selector5 : Selector  InputPortWidth=2  IndexOptions=Index vector (dialog)  Indices=2  OutputSizes=1
  State-Space x : StateSpace  A=A  B=B  C=C  D=D  InitialCondition=XIV
  State-Space y : StateSpace  A=A  B=B  C=C  D=D  InitialCondition=XIV
  state : Outport
  wires:
  vol/1 -> Selector3/1, Selector5/1
  Selector3/1 -> State-Space x/1
  Selector5/1 -> State-Space y/1
  State-Space x/1 -> Matrix Concatenate1/1
  State-Space y/1 -> Matrix Concatenate1/2
  Matrix Concatenate1/1 -> state/1

== system Ballbot_System_LQR/Controller/Controller/State/Cal_psidot/Update_gyro_offset ==
  note: Low Path Filter
      |   gyro_offset_u = (1 - a_gd) * gyro_read + a_gd * gyro_offset
  gyro : Inport
  gyro_offset : Inport  Port=2
  Delay : Delay  DelayLength=1  InitialConditionSource=Input port
      settings: InputPortMap=u0,p4
  Gain : Gain  Gain=1 - a_gd
  Gain1 : Gain  Gain=a_gd
  Sum : Sum  Inputs=|++
  gyro_offset_u : Outport
  wires:
  gyro/1 -> Gain/1
  Gain/1 -> Sum/1
  Gain1/1 -> Sum/2
  Sum/1 -> Delay/1, gyro_offset_u/1
  Delay/1 -> Gain1/1
  gyro_offset/1 -> Delay/2
